simulink model "simFC"  (R2023b)
settings: Solver=ode15s  StartTime=0.0  StopTime=100.0  RelTol=1e-3
values from neighbouring files (symbols this model uses):
  beta = .1    (= 0.1)    [runFC.m]
  D_d = eye(6)*3    [runFC.m]
  dragcoeff = [C_d_1, C_d_4, C_d_C, C_d_L, beta, gamma]    [runFC.m]
  G_d = eye(6)*0.5    [runFC.m]
  gamma = .1    (= 0.1)    [runFC.m]
  K_D = blkdiag(eye(3),eye(3),eye(9))*500    [runFC.m]
  K_DI = diag([0.5 0.5 0.5 0.1 0.1 0.1])*2    [runFC.m]
  K_FI = diag([0.5 0.5 0.5 0.3 0.3 0.3])/1.05    [runFC.m]
  K_FP = diag([1 1 1 0.2 0.2 0.2])/1.3    [runFC.m]
  K_II = diag([0.2 0.2 0.2 0.15 0.15 0.15]*20)    [runFC.m]
  K_P = blkdiag(eye(3),eye(3),eye(9)*30)    [runFC.m]
  K_SI = diag([1 1 1 0.2 0.2 0.2])*30    [runFC.m]
  Lambda = blkdiag(eye(3)*40,eye(3)*40,eye(9)*40)    [runFC.m]
  M_d = eye(6)*4    [runFC.m]
  pos_init = [-0.02 (2*0.77*cos(pi/4)+1) 0]    [runFC.m]
  quat_init = eul2quat([0 0 pi],'XYZ')    [runFC.m]
  theta_init = [0 pi/4 0 pi/4 pi/4 0 pi/4 0 0]    [runFC.m]
  x_init = [pos_init quat_init theta_init zeta_init]'    [runFC.m]
undefined symbols (not defined in the file or in its folder): pp, snake
libraries: cstblocks x3, dspindex x2
settings Model: Creator=sarava  LastModifiedBy=asker
settings SolverCC: AlgebraicLoopSolver=TrustRegion
settings DataIOCC: ReturnWorkspaceOutputs=off
settings DebuggingCC: UnconnectedInputMsg=warning  UnconnectedOutputMsg=warning  UnconnectedLineMsg=warning  ArithmeticOperatorsInVariantConditions=warning
settings ModelReferenceCC: EnableRefExpFcnMdlSchedulingChecks=on
settings SFSimCC: SimUseLocalCustomCode=off  CustomCodeUndefinedFunction=UseInterfaceOnly
settings RTWCC: RTWUseLocalCustomCode=off

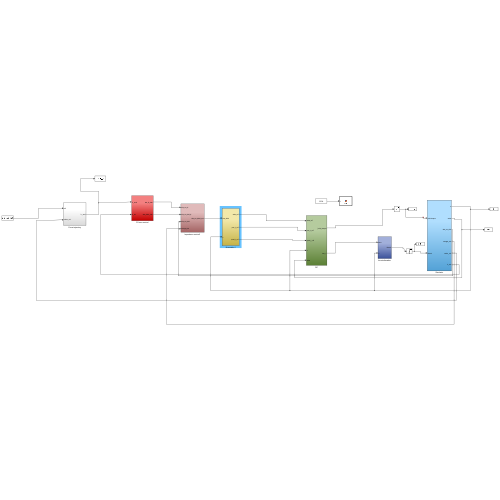
[thumbnail: Simulink's stored preview of the top-level diagram]
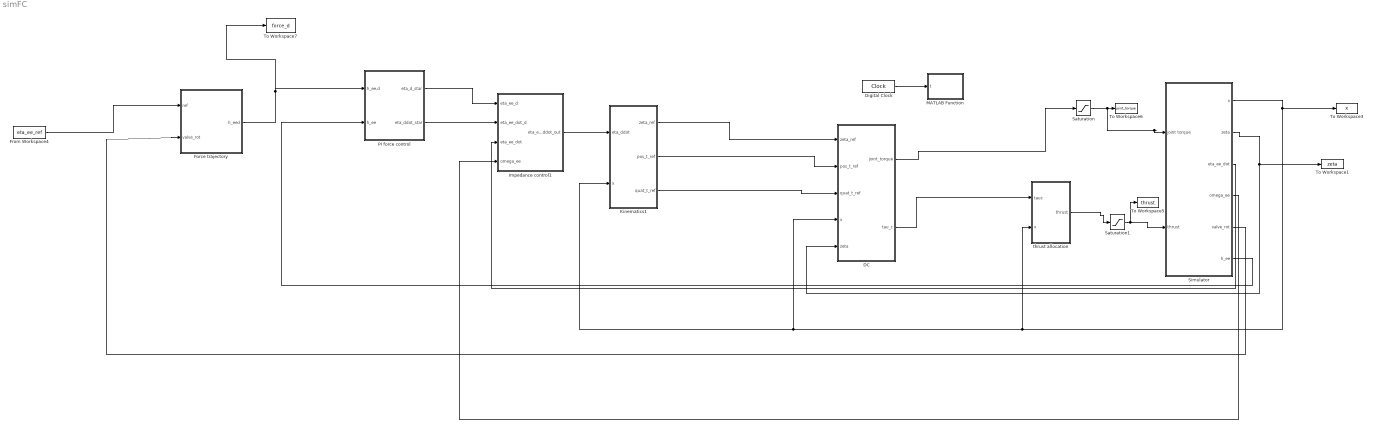
== system simFC ==
  DC : Subsystem
  Digital Clock : DigitalClock
  Force trajectory : Subsystem
  From Workspace4 : FromWorkspace  VariableName=eta_ee_ref
  Impedance control1 : Subsystem
  Kinematics1 : Subsystem
  MATLAB Function : MATLAB Function  TreatAsAtomicUnit=on
  PI force control : Subsystem
  Saturation : Saturate  UpperLimit=8  LowerLimit=-2  ZeroCross=off
  Saturation1 : Saturate  UpperLimit=5  LowerLimit=-5  ZeroCross=off
  Simulator : Subsystem
  To Workspace1 : ToWorkspace  VariableName=zeta  SaveFormat=Timeseries  SampleTime=-1
  To Workspace3 : ToWorkspace  VariableName=x  SaveFormat=Timeseries  SampleTime=-1
  To Workspace5 : ToWorkspace  VariableName=thrust  SaveFormat=Timeseries  SampleTime=-1
  To Workspace6 : ToWorkspace  VariableName=joint_torque  SaveFormat=Timeseries  SampleTime=-1
  To Workspace7 : ToWorkspace  VariableName=force_d  SaveFormat=Timeseries  SampleTime=-1
  thrust allocation : Subsystem
  wires:
  Digital Clock/1 -> MATLAB Function/1(t)
  Simulator/4(omega_ee) -> Impedance control1/4(omega_ee)
  Simulator/1(x) -> To Workspace3/1, thrust allocation/2("x "), Kinematics1/2(x), DC/4(x)
  DC/1(joint_torque) -> Saturation/1
  Impedance control1/1(eta_ee_ddot_out) -> Kinematics1/1(eta_ddot)
  thrust allocation/1(thrust) -> Saturation1/1
  Kinematics1/2(pos_t_ref) -> DC/2(pos_t_ref)
  Saturation1/1 -> To Workspace5/1, Simulator/2(thrust)
  Simulator/2(zeta) -> DC/5("zeta "), To Workspace1/1
  DC/2(tau_c) -> thrust allocation/1("tauc ")
  Kinematics1/3(quat_t_ref) -> DC/3(quat_t_ref)
  Saturation/1 -> Simulator/1(joint torque), To Workspace6/1
  Kinematics1/1(zeta_ref) -> DC/1(zeta_ref)
  Simulator/3(eta_ee_dot) -> Impedance control1/3(eta_ee_dot)
  Force trajectory/1(h_eed) -> To Workspace7/1, PI force control/1(h_ee,d)
  From Workspace4/1 -> Force trajectory/1(ref)
  Simulator/5(valve_rot) -> Force trajectory/2(valve_rot)
  Simulator/6(h_ee) -> PI force control/2(h_ee)
  PI force control/1(eta_d_star) -> Impedance control1/1(eta_ee_d)
  PI force control/2(eta_ddot_star) -> Impedance control1/2(eta_ee_dot_d)

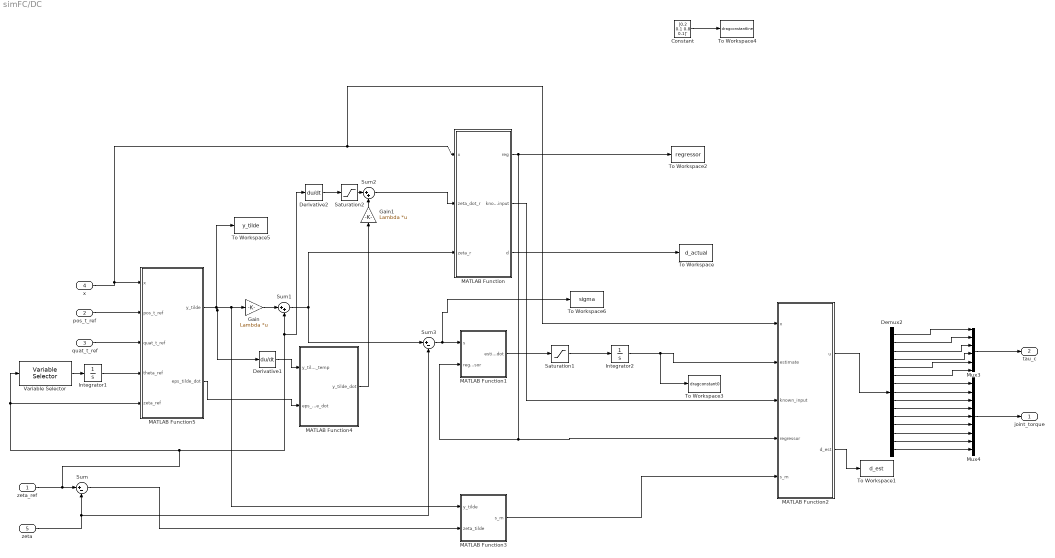
== system simFC/DC ==
  zeta_ref : Inport
  pos_t_ref : Inport  Port=2
  quat_t_ref : Inport  Port=3
  x : Inport  Port=4
  "zeta " : Inport  Port=5
  Constant : Constant  Value=[0.2 0.1 0.8 0.1]'
  Demux2 : Demux  Outputs=15
  Derivative1 : Derivative  CoefficientInTFapproximation=10
  Derivative2 : Derivative  CoefficientInTFapproximation=10
  Gain : Gain  Gain=Lambda  Multiplication=Matrix(K*u) (u vector)
  Gain1 : Gain  Gain=Lambda  Multiplication=Matrix(K*u) (u vector)
  Integrator1 : Integrator  InitialCondition=theta_init
  Integrator2 : Integrator  InitialCondition=[0 0 0 0]'
  MATLAB Function : MATLAB Function  TreatAsAtomicUnit=on
  MATLAB Function1 : MATLAB Function  TreatAsAtomicUnit=on
  MATLAB Function2 : MATLAB Function  TreatAsAtomicUnit=on
  MATLAB Function3 : MATLAB Function  TreatAsAtomicUnit=on
  MATLAB Function4 : MATLAB Function  TreatAsAtomicUnit=on
  MATLAB Function5 : MATLAB Function  TreatAsAtomicUnit=on
  Mux3 : Mux  Inputs=6
  Mux4 : Mux  Inputs=9
  Saturation1 : Saturate  UpperLimit=50  LowerLimit=-50  ZeroCross=off
  Saturation2 : Saturate  UpperLimit=20  LowerLimit=-20  ZeroCross=off
  Sum : Sum  Inputs=|+-
  Sum1 : Sum  Inputs=|++
  Sum2 : Sum  Inputs=|++
  Sum3 : Sum  Inputs=|+-
  To Workspace : ToWorkspace  VariableName=d_actual  SaveFormat=Timeseries  SampleTime=-1
  To Workspace1 : ToWorkspace  VariableName=d_est  SaveFormat=Timeseries  SampleTime=-1
  To Workspace2 : ToWorkspace  VariableName=regressor  SaveFormat=Timeseries  SampleTime=-1
  To Workspace3 : ToWorkspace  VariableName=dragconstant0  SaveFormat=Timeseries  SampleTime=-1
  To Workspace4 : ToWorkspace  VariableName=dragconstantline  SaveFormat=Timeseries  SampleTime=-1
  To Workspace5 : ToWorkspace  VariableName=y_tilde  SaveFormat=Timeseries  SampleTime=-1
  To Workspace6 : ToWorkspace  VariableName=sigma  SaveFormat=Timeseries  SampleTime=-1
  Variable Selector : dspindex/Variable Selector  NumInputs=1  rowsOrCols=Rows  IdxMode=Fixed  Elements=7:15  ZerOneIdxMode=One-based  errmode=Clip Index  FillMode=on  FillValues=0
  joint_torque : Outport  VectorParamsAs1DForOutWhenUnconnected=off
  tau_c : Outport  Port=2  VectorParamsAs1DForOutWhenUnconnected=off
  wires:
  x/1 -> MATLAB Function/1(x), MATLAB Function2/1(x), MATLAB Function5/1(x)
  pos_t_ref/1 -> MATLAB Function5/2(pos_t_ref)
  quat_t_ref/1 -> MATLAB Function5/3(quat_t_ref)
  zeta_ref/1 -> Derivative2/1, Sum1/2, Variable Selector/1, MATLAB Function5/5(zeta_ref), Sum/1
  "zeta "/1 -> Sum3/2, Sum/2
  Integrator1/1 -> MATLAB Function5/4(theta_ref)
  MATLAB Function5/1(y_tilde) -> MATLAB Function3/1(y_tilde), Gain/1, Derivative1/1, To Workspace5/1
  Gain/1 -> Sum1/1
  Sum1/1 -> Sum3/1, MATLAB Function/3(zeta_r)
  Saturation1/1 -> Integrator2/1
  MATLAB Function1/1(estimate_dot) -> Saturation1/1
  MATLAB Function3/1(s_m) -> MATLAB Function2/5(s_m)
  MATLAB Function2/1(u) -> Demux2/1
  Demux2/14 -> Mux4/8
  Demux2/4 -> Mux3/4
  Demux2/5 -> Mux3/5
  Demux2/12 -> Mux4/6
  Demux2/2 -> Mux3/2
  Demux2/9 -> Mux4/3
  Demux2/3 -> Mux3/3
  Demux2/13 -> Mux4/7
  Demux2/8 -> Mux4/2
  Demux2/6 -> Mux3/6
  Demux2/10 -> Mux4/4
  Demux2/7 -> Mux4/1
  Demux2/11 -> Mux4/5
  Demux2/1 -> Mux3/1
  Mux4/1 -> joint_torque/1
  Mux3/1 -> tau_c/1
  Variable Selector/1 -> Integrator1/1
  Integrator2/1 -> To Workspace3/1, MATLAB Function2/2(estimate)
  MATLAB Function/2(known_input) -> MATLAB Function2/3(known_input)
  MATLAB Function/1(reg) -> MATLAB Function1/2(regressor), MATLAB Function2/4(regressor), To Workspace2/1
  MATLAB Function5/2(eps_tilde_dot) -> MATLAB Function4/2(eps_tilde_dot)
  Derivative1/1 -> MATLAB Function4/1(y_tilde_dot_temp)
  MATLAB Function4/1(y_tilde_dot) -> Gain1/1
  Derivative2/1 -> Saturation2/1
  Saturation2/1 -> Sum2/1
  Gain1/1 -> Sum2/2
  Sum3/1 -> To Workspace6/1, MATLAB Function1/1(s)
  Sum2/1 -> MATLAB Function/2(zeta_dot_r)
  Sum/1 -> MATLAB Function3/2(zeta_tilde)
  MATLAB Function/3(d) -> To Workspace/1
  MATLAB Function2/2(d_est) -> To Workspace1/1
  Constant/1 -> To Workspace4/1
  Demux2/15 -> Mux4/9

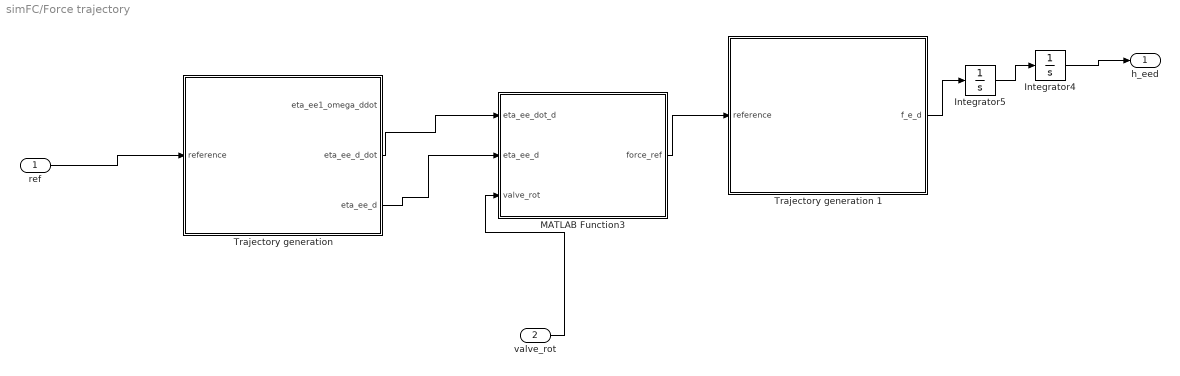
== system simFC/Force trajectory ==
  ref : Inport
  valve_rot : Inport  Port=2
  Integrator4 : Integrator  InitialCondition=[0 0 0 0 0 0]'
  Integrator5 : Integrator  InitialCondition=[0 0 0 0 0 0]'
  MATLAB Function3 : MATLAB Function  TreatAsAtomicUnit=on
  "Trajectory generation " : Subsystem
  Trajectory generation 1 : Subsystem
  h_eed : Outport  VectorParamsAs1DForOutWhenUnconnected=off
  wires:
  valve_rot/1 -> MATLAB Function3/3(valve_rot)
  ref/1 -> "Trajectory generation "/1(reference)
  "Trajectory generation "/2(eta_ee_d_dot) -> MATLAB Function3/1(eta_ee_dot_d)
  Trajectory generation 1/1(f_e_d) -> Integrator5/1
  Integrator5/1 -> Integrator4/1
  "Trajectory generation "/3(eta_ee_d) -> MATLAB Function3/2(eta_ee_d)
  Integrator4/1 -> h_eed/1
  MATLAB Function3/1(force_ref) -> Trajectory generation 1/1(reference)

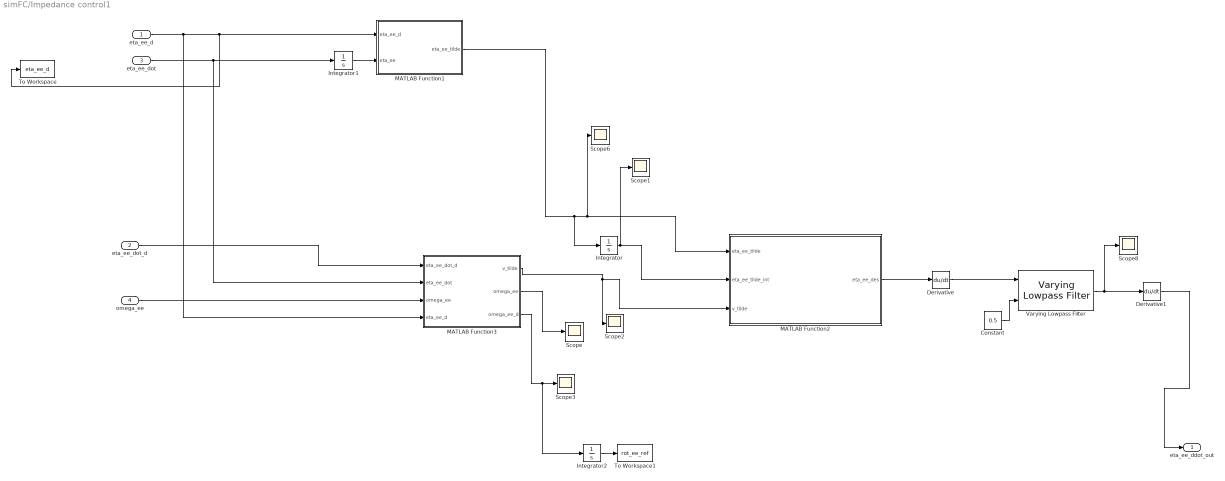
== system simFC/Impedance control1 ==
  eta_ee_d : Inport
  eta_ee_dot_d : Inport  Port=2
  eta_ee_dot : Inport  Port=3
  omega_ee : Inport  Port=4
  Constant : Constant  Value=0.5
  Derivative : Derivative
  Derivative1 : Derivative
  Integrator : Integrator
  Integrator1 : Integrator
  Integrator2 : Integrator
  MATLAB Function1 : MATLAB Function  TreatAsAtomicUnit=on
  MATLAB Function2 : MATLAB Function  TreatAsAtomicUnit=on
  MATLAB Function3 : MATLAB Function  TreatAsAtomicUnit=on
  Scope{,1..3,6,8} (6 alike) : Scope
  To Workspace : ToWorkspace  VariableName=eta_ee_d  SaveFormat=Timeseries  SampleTime=-1
  To Workspace1 : ToWorkspace  VariableName=rot_ee_ref  SaveFormat=Timeseries  SampleTime=-1
  Varying Lowpass Filter : cstblocks/Linear Parameter Varying/Varying Lowpass Filter  N=1
  eta_ee_ddot_out : Outport  VectorParamsAs1DForOutWhenUnconnected=off
  wires:
  eta_ee_d/1 -> MATLAB Function3/4(eta_ee_d), To Workspace/1, MATLAB Function1/1(eta_ee_d)
  eta_ee_dot_d/1 -> MATLAB Function3/1(eta_ee_dot_d)
  eta_ee_dot/1 -> Integrator1/1, MATLAB Function3/2(eta_ee_dot)
  omega_ee/1 -> MATLAB Function3/3("omega_ee ")
  MATLAB Function3/1(v_tilde) -> MATLAB Function2/3(v_tilde), Scope2/1
  MATLAB Function1/1(eta_ee_tilde) -> Integrator/1, Scope6/1, MATLAB Function2/1(eta_ee_tilde)
  Integrator/1 -> Scope1/1, MATLAB Function2/2(eta_ee_tilde_int)
  MATLAB Function3/2(omega_ee) -> Scope/1
  MATLAB Function2/1(eta_ee_des) -> Derivative/1
  Integrator1/1 -> MATLAB Function1/2(eta_ee)
  MATLAB Function3/3(omega_ee_d) -> Integrator2/1, Scope3/1
  Constant/1 -> Varying Lowpass Filter/2
  Derivative/1 -> Varying Lowpass Filter/1
  Varying Lowpass Filter/1 -> Derivative1/1, Scope8/1
  Integrator2/1 -> To Workspace1/1
  Derivative1/1 -> eta_ee_ddot_out/1

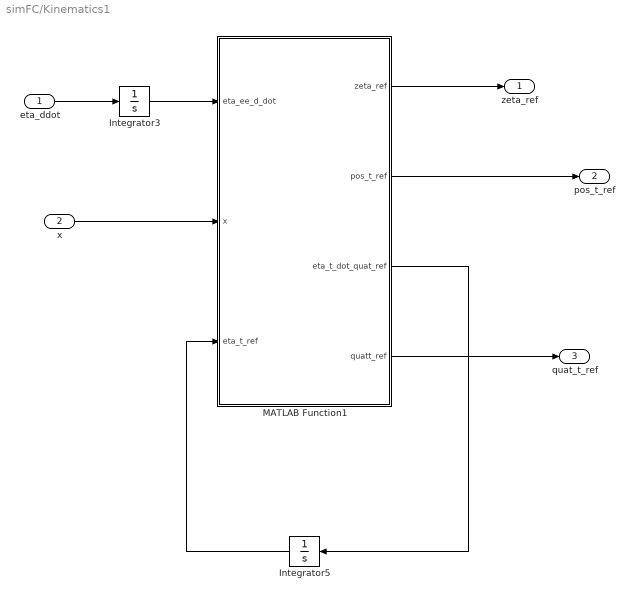
== system simFC/Kinematics1 ==
  eta_ddot : Inport
  x : Inport  Port=2
  Integrator3 : Integrator
  Integrator5 : Integrator  InitialCondition=[pos_init quat_init]'
  MATLAB Function1 : MATLAB Function  TreatAsAtomicUnit=on
  zeta_ref : Outport  VectorParamsAs1DForOutWhenUnconnected=off
  pos_t_ref : Outport  Port=2  VectorParamsAs1DForOutWhenUnconnected=off
  quat_t_ref : Outport  Port=3  VectorParamsAs1DForOutWhenUnconnected=off
  wires:
  x/1 -> MATLAB Function1/2(x)
  MATLAB Function1/1(zeta_ref) -> zeta_ref/1
  MATLAB Function1/2(pos_t_ref) -> pos_t_ref/1
  eta_ddot/1 -> Integrator3/1
  Integrator3/1 -> MATLAB Function1/1(eta_ee_d_dot)
  MATLAB Function1/3(eta_t_dot_quat_ref) -> Integrator5/1
  Integrator5/1 -> MATLAB Function1/3(eta_t_ref)
  MATLAB Function1/4(quatt_ref) -> quat_t_ref/1

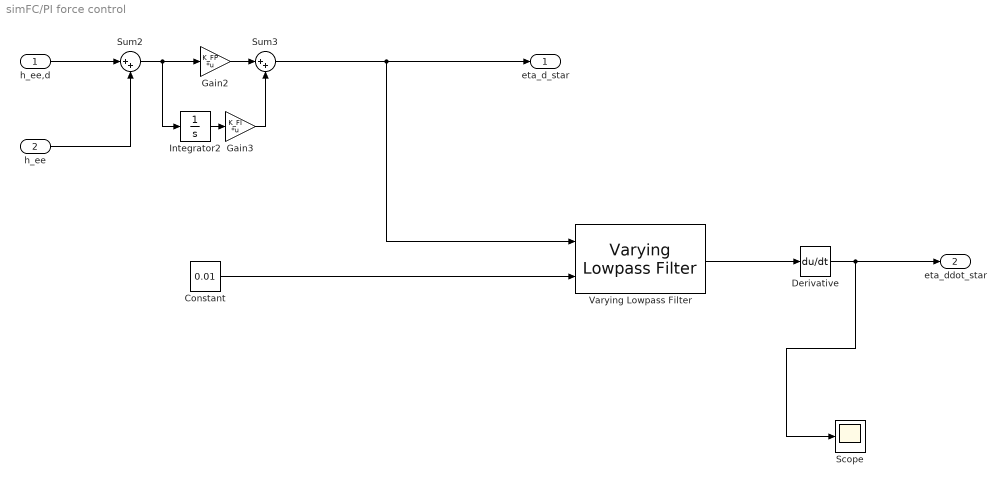
== system simFC/PI force control ==
  h_ee,d : Inport
  h_ee : Inport  Port=2
  Constant : Constant  Value=0.01
  Derivative : Derivative
  Gain2 : Gain  Gain=K_FP  Multiplication=Matrix(K*u)
  Gain3 : Gain  Gain=K_FI  Multiplication=Matrix(K*u)
  Integrator2 : Integrator
  Scope : Scope
  Sum2 : Sum  Inputs=|++
  Sum3 : Sum  Inputs=|++
  Varying Lowpass Filter : cstblocks/Linear Parameter Varying/Varying Lowpass Filter  N=1
  eta_d_star : Outport  VectorParamsAs1DForOutWhenUnconnected=off
  eta_ddot_star : Outport  Port=2  VectorParamsAs1DForOutWhenUnconnected=off
  wires:
  Constant/1 -> Varying Lowpass Filter/2
  Sum3/1 -> eta_d_star/1, Varying Lowpass Filter/1
  Gain3/1 -> Sum3/2
  Integrator2/1 -> Gain3/1
  Sum2/1 -> Integrator2/1, Gain2/1
  Gain2/1 -> Sum3/1
  h_ee/1 -> Sum2/2
  h_ee,d/1 -> Sum2/1
  Varying Lowpass Filter/1 -> Derivative/1
  Derivative/1 -> eta_ddot_star/1, Scope/1

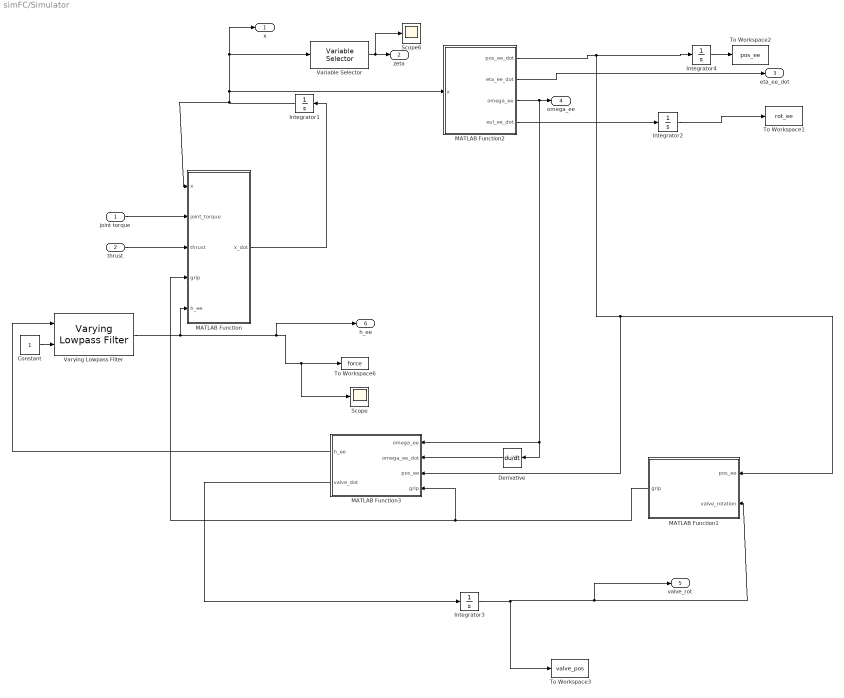
== system simFC/Simulator ==
  joint torque : Inport
  thrust : Inport  Port=2
  Constant : Constant
  Derivative : Derivative
  Integrator1 : Integrator  InitialCondition=x_init
  Integrator2 : Integrator
  Integrator3 : Integrator
  Integrator4 : Integrator
  MATLAB Function : MATLAB Function  TreatAsAtomicUnit=on
  MATLAB Function1 : MATLAB Function  TreatAsAtomicUnit=on
  MATLAB Function2 : MATLAB Function  TreatAsAtomicUnit=on
  MATLAB Function3 : MATLAB Function  TreatAsAtomicUnit=on
  Scope : Scope
  Scope6 : Scope
  To Workspace1 : ToWorkspace  VariableName=rot_ee  SaveFormat=Timeseries  SampleTime=-1
  To Workspace2 : ToWorkspace  VariableName=pos_ee  SaveFormat=Timeseries  SampleTime=-1
  To Workspace3 : ToWorkspace  VariableName=valve_pos  SaveFormat=Timeseries  SampleTime=-1
  To Workspace6 : ToWorkspace  VariableName=force  SaveFormat=Timeseries  SampleTime=-1
  Variable Selector : dspindex/Variable Selector  NumInputs=1  rowsOrCols=Rows  IdxMode=Fixed  Elements=17:31  ZerOneIdxMode=One-based  errmode=Clip Index  FillMode=on  FillValues=0
  Varying Lowpass Filter : cstblocks/Linear Parameter Varying/Varying Lowpass Filter  N=1
  x : Outport  VectorParamsAs1DForOutWhenUnconnected=off
  zeta : Outport  Port=2  VectorParamsAs1DForOutWhenUnconnected=off
  eta_ee_dot : Outport  Port=3  VectorParamsAs1DForOutWhenUnconnected=off
  omega_ee : Outport  Port=4  VectorParamsAs1DForOutWhenUnconnected=off
  valve_rot : Outport  Port=5  VectorParamsAs1DForOutWhenUnconnected=off
  h_ee : Outport  Port=6  VectorParamsAs1DForOutWhenUnconnected=off
  wires:
  joint torque/1 -> MATLAB Function/2(joint_torque)
  thrust/1 -> MATLAB Function/3(thrust)
  Variable Selector/1 -> Scope6/1, zeta/1
  MATLAB Function2/1(pos_ee_dot) -> Integrator4/1, MATLAB Function3/3(pos_ee), MATLAB Function1/1(pos_ee)
  MATLAB Function/1(x_dot) -> Integrator1/1
  Integrator1/1 -> Variable Selector/1, x/1, MATLAB Function2/1(x), MATLAB Function/1(x)
  MATLAB Function2/2(eta_ee_dot) -> eta_ee_dot/1
  MATLAB Function2/3(omega_ee) -> Derivative/1, MATLAB Function3/1(omega_ee), omega_ee/1
  Integrator2/1 -> To Workspace1/1
  MATLAB Function3/1(h_ee) -> Varying Lowpass Filter/1
  MATLAB Function1/1(grip) -> MATLAB Function3/4(grip), MATLAB Function/4(grip)
  MATLAB Function3/2(valve_dot) -> Integrator3/1
  Integrator3/1 -> valve_rot/1, MATLAB Function1/2(valve_rotation), To Workspace3/1
  Derivative/1 -> MATLAB Function3/2(omega_ee_dot)
  Varying Lowpass Filter/1 -> MATLAB Function/5(h_ee), h_ee/1, Scope/1, To Workspace6/1
  Constant/1 -> Varying Lowpass Filter/2
  Integrator4/1 -> To Workspace2/1
  MATLAB Function2/4(eul_ee_dot) -> Integrator2/1

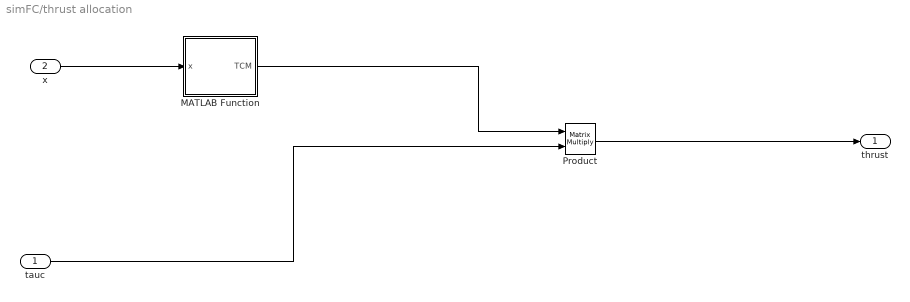
== system simFC/thrust allocation ==
  "tauc " : Inport
  "x " : Inport  Port=2
  MATLAB Function : MATLAB Function  TreatAsAtomicUnit=on
  Product : Product  Multiplication=Matrix(*)
  thrust : Outport  VectorParamsAs1DForOutWhenUnconnected=off
  wires:
  "x "/1 -> MATLAB Function/1(x)
  MATLAB Function/1(TCM) -> Product/1
  "tauc "/1 -> Product/2
  Product/1 -> thrust/1

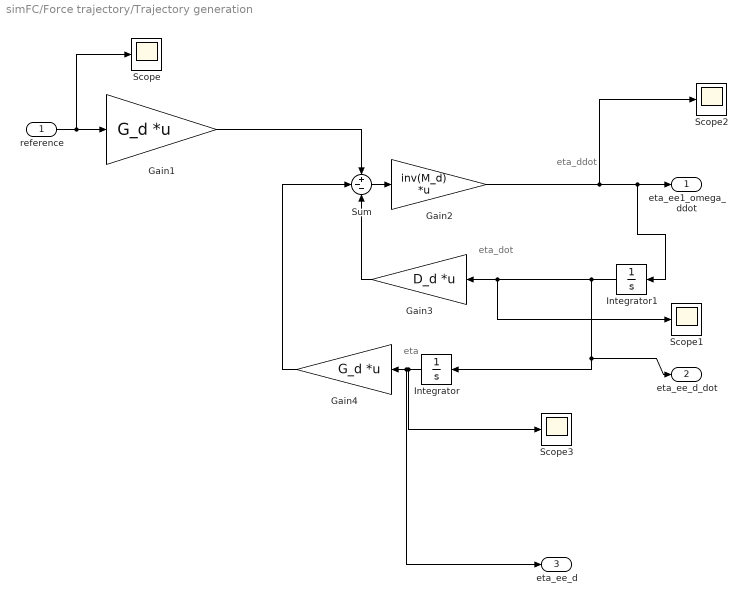
== system simFC/Force trajectory/Trajectory generation  ==
  note: eta_dot
  note: eta
  note: eta_ddot
  reference : Inport
  Gain1 : Gain  Gain=G_d  Multiplication=Matrix(K*u) (u vector)
  Gain2 : Gain  Gain=inv(M_d)  Multiplication=Matrix(K*u) (u vector)
  Gain3 : Gain  Gain=D_d  Multiplication=Matrix(K*u) (u vector)
  Gain4 : Gain  Gain=G_d  Multiplication=Matrix(K*u) (u vector)
  Integrator : Integrator  InitialCondition=[0 0 0 0 0 0]'
  Integrator1 : Integrator  InitialCondition=[0 0 0 0 0 0]'
  Scope{,1..3} (4 alike) : Scope
  Sum : Sum  Inputs=+--
  eta_ee1_omega_ddot : Outport  VectorParamsAs1DForOutWhenUnconnected=off
  eta_ee_d_dot : Outport  Port=2  VectorParamsAs1DForOutWhenUnconnected=off
  eta_ee_d : Outport  Port=3  VectorParamsAs1DForOutWhenUnconnected=off
  wires:
  Gain2/1 -> Scope2/1, eta_ee1_omega_ddot/1, Integrator1/1
  Gain1/1 -> Sum/1
  Sum/1 -> Gain2/1
  reference/1 -> Scope/1, Gain1/1
  Integrator1/1 -> eta_ee_d_dot/1, Integrator/1, Scope1/1, Gain3/1
  Integrator/1 -> Scope3/1, eta_ee_d/1, Gain4/1
  Gain3/1 -> Sum/3
  Gain4/1 -> Sum/2

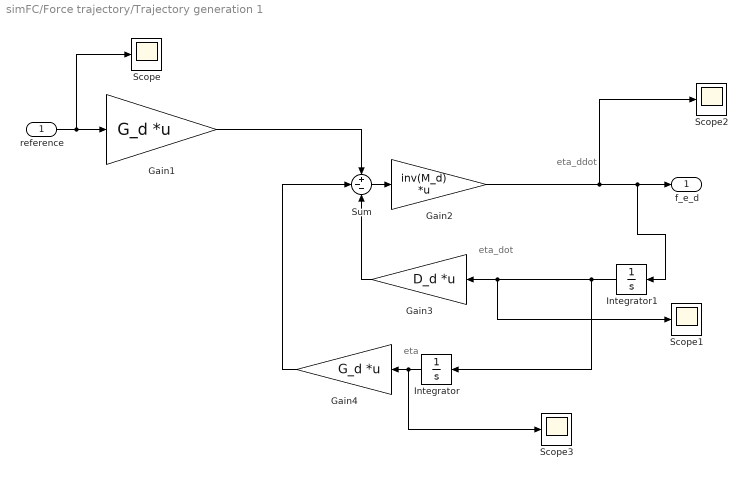
== system simFC/Force trajectory/Trajectory generation 1 ==
  note: eta_dot
  note: eta
  note: eta_ddot
  reference : Inport
  Gain1 : Gain  Gain=G_d  Multiplication=Matrix(K*u) (u vector)
  Gain2 : Gain  Gain=inv(M_d)  Multiplication=Matrix(K*u) (u vector)
  Gain3 : Gain  Gain=D_d  Multiplication=Matrix(K*u) (u vector)
  Gain4 : Gain  Gain=G_d  Multiplication=Matrix(K*u) (u vector)
  Integrator : Integrator  InitialCondition=[0 0 0 0 0 0]'
  Integrator1 : Integrator  InitialCondition=[0 0 0 0 0 0]'
  Scope{,1..3} (4 alike) : Scope
  Sum : Sum  Inputs=+--
  f_e_d : Outport  VectorParamsAs1DForOutWhenUnconnected=off
  wires:
  Gain2/1 -> Scope2/1, f_e_d/1, Integrator1/1
  Gain1/1 -> Sum/1
  Sum/1 -> Gain2/1
  reference/1 -> Scope/1, Gain1/1
  Integrator1/1 -> Integrator/1, Scope1/1, Gain3/1
  Integrator/1 -> Scope3/1, Gain4/1
  Gain3/1 -> Sum/3
  Gain4/1 -> Sum/2

== matlab function simFC/Force trajectory/MATLAB Function3 ==
  data: eta_ee_dot_d input; eta_ee_d input; force_ref output; valve_rot input
function force_ref = fcn(eta_ee_dot_d,  eta_ee_d, valve_rot)

eta_ee2_dot_d=eta_ee_dot_d(4:6);


phi=eta_ee_d(4);
theta=eta_ee_d(5);
psi=eta_ee_d(6);

J=[1 0 -sin(theta); 0 cos(theta) cos(theta)*sin(phi); 0 -sin(phi) cos(theta)*cos(phi)];
R=rotx(rad2deg(phi))*roty(rad2deg(theta))*rotz(rad2deg(psi));

omega_ee_d=500*R*J*eta_ee2_dot_d;
if valve_rot<=pi/4
force_ref=[0; 0; 0; omega_ee_d(1); 0; 0];
else
    force_ref=[0; 0; 0; 0; 0; 0];
end

== matlab function simFC/DC/MATLAB Function4 ==
  data: y_tilde_dot_temp input; eps_tilde_dot input; y_tilde_dot output
function y_tilde_dot = calc_estdot(y_tilde_dot_temp,eps_tilde_dot)

y_tilde_dot=[y_tilde_dot_temp(1:3);eps_tilde_dot;y_tilde_dot_temp(7:15)];
end

== matlab function simFC/Simulator/MATLAB Function3 ==
  data: omega_ee input; omega_ee_dot input; pos_ee input; h_ee output size=6; grip input; valve_dot output; valve_pos parameter
function [h_ee,valve_dot]= vent(omega_ee,omega_ee_dot,pos_ee,grip,valve_pos)
x=pos_ee(1);
xe=valve_pos(1);
J_v=3  ;
my_v=500;
if  grip==1
    my_ee=[J_v*omega_ee_dot(1)+my_v*omega_ee(1); 0;0];
else
    my_ee=[0 0 0]';
end
f_ee=[0 0 0]';


if (x-xe)>0
    f_ee(1)=20*(x-xe);
end



h_ee=-[f_ee;my_ee];
%h_ee=[0 0 0 0 0 0]';

if grip==true
    valve_dot=omega_ee(1);
else
    valve_dot=0;
end
end

== matlab function simFC/Simulator/MATLAB Function1 ==
  data: pos_ee input; valve_rotation input; grip output; valve_pos parameter
function grip = vent(pos_ee,valve_rotation,valve_pos)
grip=false;
if abs(pos_ee-valve_pos)<0.3
    grip=true;
%      if valve_rotation(1)>pi/4
%          grip=false;
%      end
end
error=pos_ee-valve_pos;
grip=true;
end

== matlab function simFC/DC/MATLAB Function ==
  data: x input; zeta_dot_r input; reg output; known_input output; snake parameter; pp parameter; gamma parameter; beta parameter; zeta_r input; d output
function [reg, known_input,d] = regressor(x,zeta_dot_r,snake,pp, gamma, beta, zeta_r)

quat      =  x(4:7);
theta     =  x(8 : 6+snake.n);
zeta      =  x(7+snake.n : 11+2*snake.n);
[R, J]    =  comp_rot_jac(quat,theta,snake);
[c,d,g,D] = comp_cdg_adaptiv(J,R,theta,snake,pp,beta,gamma,zeta,zeta_r);
M = comp_mass(J,snake);




drag_matrix=zeros(15,4);
for i=1:snake.n
 drag_matrix=drag_matrix+J(:,:,i)'*D(:,:,i);
end



known_input= M*zeta_dot_r+c+g;

reg=drag_matrix;


end

== matlab function simFC/DC/MATLAB Function1 ==
  data: s input; regressor input; estimate_dot output; K_theta parameter
function estimate_dot = calc_estdot(s,regressor,K_theta)


estimate_dot=inv(K_theta)*regressor'*s;

end

== matlab function simFC/DC/MATLAB Function2 ==
  data: x input; estimate input; known_input input; regressor input; u output; s_m input; K_D parameter; snake parameter; d_est output
function [u,d_est]= input(x,estimate,known_input,regressor,s_m, K_D,snake)

quat      =  x(4:7);
theta     =  x(8 : 6+snake.n);

[~, J]    =  comp_rot_jac(quat,theta,snake);


B=comp_TCM(J,snake);
B_u=[eye(6,6) zeros(6,9); B(7:end,:)*pinv(B(1:6,:)) eye(9)];
d_est=regressor*estimate;
u=pinv(B_u)*(K_D*s_m+known_input+regressor*estimate);
end

== matlab function simFC/DC/MATLAB Function3 ==
  data: y_tilde input; zeta_tilde input; s_m output; Lambda parameter; K_D parameter; K_P parameter
function s_m = calc_estdot(y_tilde, zeta_tilde, Lambda, K_D, K_P)


s_m=zeta_tilde+Lambda*y_tilde + inv(K_D)*K_P*y_tilde;
end

== matlab function simFC/DC/MATLAB Function5 ==
  data: x input; y_tilde output; pos_t_ref input size=3; quat_t_ref input size=4; theta_ref input; eps_tilde_dot output; zeta_ref input
function [y_tilde,eps_tilde_dot] = dyn(x,pos_t_ref, quat_t_ref, theta_ref, zeta_ref)
pos_t=x(1:3);
quat      =  x(4:7);
theta     =  x(8 : 16);
zeta     =  x( 17: 31);

theta_tilde=theta_ref-theta;

pos_tilde=quat2rotm(quat')*(pos_t_ref-pos_t);
pos_tilde2=RotQ(quat)*(pos_t_ref-pos_t);



quat_tilde=quat(1)*quat_t_ref(2:4)-quat_t_ref(1)*quat(2:4)+cross(quat_t_ref(2:4),quat(2:4));
eta_tilde = quat(1) * quat_t_ref (1) + quat_t_ref(2:4)'*quat(2:4);
if eta_tilde < 0
quat_tilde = - quat_tilde ;
end


y_tilde=[pos_tilde;quat_tilde; theta_tilde];

out=pos_t_ref-pos_t;
nu2_tilde=zeta_ref(4:6)-zeta(4:6);
eps_tilde_dot=0.5*eta_tilde*nu2_tilde + 0.5*skew(quat_tilde)*nu2_tilde;

end

== matlab function simFC/Impedance control1/MATLAB Function1 ==
  data: eta_ee_tilde output; eta_ee_d input; eta_ee input
function eta_ee_tilde = fcn(eta_ee_d, eta_ee)

eta_ee1_d=eta_ee_d(1:3);
eta_ee1=eta_ee(1:3);

quat_ee_d=eul2quat(eta_ee_d(4:6)','XYZ')';
quat_ee=eul2quat(eta_ee(4:6)','XYZ')';

quat_error=quat_ee(1)*quat_ee_d(2:4)-quat_ee_d(1)*quat_ee(2:4)-cross(quat_ee_d(2:4),quat_ee(2:4));

eta_ee_tilde=[eta_ee1_d-eta_ee1;quat_error];

== matlab function simFC/Impedance control1/MATLAB Function2 ==
  data: eta_ee_tilde input; eta_ee_des output; eta_ee_tilde_int input; v_tilde input; K_SI parameter; K_DI parameter; K_II parameter
function eta_ee_des = fcn(eta_ee_tilde,eta_ee_tilde_int, v_tilde,K_SI, K_DI, K_II)





eta_ee_force=K_SI*eta_ee_tilde+K_DI*v_tilde+K_II*eta_ee_tilde_int;

%if grip==1
    eta_ee_des=eta_ee_force;
% else
%     eta_ee_des=eta_ee_noforce;
% end

== matlab function simFC/Impedance control1/MATLAB Function3 ==
  data: v_tilde output; eta_ee_dot_d input; eta_ee_dot input; omega_ee input; eta_ee_d input; omega_ee output; omega_ee_d output
function [v_tilde,omega_ee,omega_ee_d] = fcn(eta_ee_dot_d, eta_ee_dot,omega_ee, eta_ee_d)

eta_ee1_dot_d=eta_ee_dot_d(1:3);
eta_ee1_dot=eta_ee_dot(1:3);

eta_ee2_dot_d=eta_ee_dot_d(4:6);


phi=eta_ee_d(4);
theta=eta_ee_d(5);
psi=eta_ee_d(6);

J=[1 0 -sin(theta); 0 cos(theta) cos(theta)*sin(phi); 0 -sin(phi) cos(theta)*cos(phi)];
R=rotx(rad2deg(phi))*roty(rad2deg(theta))*rotz(rad2deg(psi));

omega_ee_d=R*J*eta_ee2_dot_d;
omega_error=omega_ee_d-omega_ee;

v_tilde=[eta_ee1_dot_d-eta_ee1_dot;omega_error];

== matlab function simFC/Simulator/MATLAB Function ==
  data: x input; x_dot output; joint_torque input; thrust input; grip input; h_ee input; pp parameter; snake parameter; dragcoeff parameter
function x_dot =  MATLAB_Function(x,joint_torque,thrust,grip,h_ee,pp , snake, dragcoeff)

pos       =  x(1:3);
quat      =  x(4:7);
theta     =  x(8 : 6+snake.n);
zeta      =  x(7+snake.n : 11+2*snake.n);
%Compute rotation matrices and jacobians
[R, J]    =  comp_rot_jac(quat,theta,snake);
[Rcdg,Jcdg]=comp_rot_jac_mcdg(quat,theta,snake);
%Compute mass matrix
M         =  comp_mass(Jcdg,snake);

%Compute relative velocity to take into account the effect of current
velc_h    =  Rcdg(:,:,1)'*pp.velc;
nu        =  zeta(1:6);
zeta(1:3) =  zeta(1:3)-velc_h;

%Compute coriolis, drag, and hydrostatic terms with the relative velocity
[c, d, g] =  comp_cdg(Jcdg,Rcdg,theta,snake,pp,dragcoeff,zeta);
%Compute the thrust-configuration matrix
B         =  comp_TCM(Jcdg,snake);

%Force
% eul_ee=rotm2eul(R(:,:,11),'XYZ')';
% Jinv=Jinv_fromeul(eul_ee);
% 
% eul_ee_ZYX=rotm2eul(R(:,:,11),'ZYX')';
% eul_ee_ZYZ=rotm2eul(R(:,:,11),'ZYZ')';
% alpha=eul_ee_ZYX(1);
% beta=eul_ee_ZYX(2);
% gamma=eul_ee_ZYX(3);

%Jinv_zyz=inv([cos(eul_ee_ZYZ(2))*sin(eul_ee_ZYZ(3)) -sin(eul_ee_ZYZ(3)) 0; cos(eul_ee_ZYZ(2))*sin(eul_ee_ZYZ(3)) cos(eul_ee_ZYZ(3)) 0; -sin(eul_ee_ZYZ(2)) 0 1]);

%Jinv_zyx=inv([-sin(beta) 0 1;cos(beta)*sin(gamma) cos(gamma) 0; cos(beta)*cos(gamma) -sin(beta) 0]);
%RJ=rotx(rad2deg(eul_ee(1)))*roty(rad2deg(eul_ee(2)))*rotz(rad2deg(eul_ee(3)));
%R(:,:,11);
J_f=[R(:,:,11) zeros(3); zeros(3) R(:,:,11)]*J(:,:,11);



%Compute the relative acceleration
if grip==1
    zeta_dot      =  M\([B [zeros(6,9); eye(9)]]*[thrust;joint_torque]-c-d-g+J_f'*h_ee);
else

    zeta_dot      =  M\([B [zeros(6,9); eye(9)]]*[thrust;joint_torque]-c-d-g);% -c-d-g
end
out=M\[B [zeros(6,9); eye(9)]]*[thrust;joint_torque];
out2=M\(-c-d-g);
%Remove the effect of current
zeta_dot(1:3) = zeta_dot(1:3)-cross(nu(4:6),velc_h);
%Compute the time derivatives of position and orientation
pos_dot   =  Rcdg(:,:,1)*nu(1:3);  
quat_dot  =  TransAngQ(quat)*nu(4:6)+1*(1-quat'*quat)*quat; 
%Assemble derivative of the state vector
x_dot = [pos_dot ; quat_dot ; zeta(7:snake.n+5) ; zeta_dot];
end

== matlab function simFC/MATLAB Function ==
  data: t input
function fcn(t)
%#codegen
coder.extrinsic('fprintf');
persistent firstTime

if isempty(firstTime)
    firstTime = false;
    fprintf('Starting Now\n');
end

fprintf('time = %.4f\n',t);

== matlab function simFC/thrust allocation/MATLAB Function ==
  data: TCM output; x input; snake parameter
function TCM = fcn(x , snake)
quat      =  x(4:7);
theta     =  x(8 : 6+snake.n);
[~, J]    =  comp_rot_jac(quat,theta,snake);
B        =  comp_TCM(J,snake);
TCM_t=B(1:6,:);
TCM=transpose(TCM_t)/(TCM_t*transpose(TCM_t));

== matlab function simFC/Simulator/MATLAB Function2 ==
  data: pos_ee_dot output; x input; snake parameter; eta_ee_dot output; omega_ee output; eul_ee_dot output
function [pos_ee_dot,eta_ee_dot, omega_ee,eul_ee_dot] = snake2points(x,snake)

   quat         = x(4:7);
   theta        = x(8 : 6+snake.n);
    zeta      =  x(7+snake.n : 11+2*snake.n);

   
   [R,J]=comp_rot_jac(quat,theta,snake);
   
   eul_ee=rotm2eul(R(:,:,11), 'XYZ')';
   Jinv=Jinv_fromeul(eul_ee);
   eta_ee_dot=[R(:,:,11) zeros(3); zeros(3) Jinv]*J(:,:,11)*zeta;
   pos_ee_dot=eta_ee_dot(1:3);
   eul_ee_dot=eta_ee_dot(4:6);
   x_ee_dot=[R(:,:,11) zeros(3); zeros(3) R(:,:,11)]*J(:,:,11)*zeta;
   omega_ee=x_ee_dot(4:6);
end

== matlab function simFC/Kinematics1/MATLAB Function1 ==
  data: eta_ee_d_dot input; x input; eta_t_ref input; zeta_ref output; snake parameter; pos_t_ref output; eta_t_dot_quat_ref output; quatt_ref output
function [zeta_ref , pos_t_ref,eta_t_dot_quat_ref, quatt_ref] = fucn(eta_ee_d_dot,x,eta_t_ref, snake)
quat      =  x(4:7);
theta     =  x(8 : 6+snake.n);
[R, J_t]    =  comp_rot_jac(quat,theta,snake);


eul_ee=rotm2eul(R(:,:,11), 'XYZ')';

Jinv=Jinv_fromeul(eul_ee);
J=[R(:,:,11) zeros(3); zeros(3) Jinv]*J_t(:,:,11);

zeta_ref=inv(diag([1 1 1 1 1 1 1 1 1 1 1 1 1 1 0.1]))*J'/(J*inv(diag([1 1 1 1 1 1 1 1 1 1 1 1 1 1 0.1]))*J'+0.0001*eye(6))*(eta_ee_d_dot);
eta_ee_ref_dot=J*zeta_ref;



quatt_ref=eta_t_ref(4:7);
pos_t_ref=eta_t_ref(1:3);
R_tail=quat2rotm(quatt_ref');

pos_t_dot   =  R_tail(:,:,1)*zeta_ref(1:3);  
quat_t_dot  =  TransAngQ(quatt_ref)*zeta_ref(4:6)+1*(1-quatt_ref'*quatt_ref)*quatt_ref; 

eta_t_dot_quat_ref=[pos_t_dot; quat_t_dot];
end
